simulink model "test_qdr_vacc2"  (Simulink 7.0)
settings: Solver=ode45  StartTime=0.0  StopTime=200000  RelTol=1e-3
libraries: xbsIndex_r4 x298, casper_library x21, xps_library x16
(part 1 of 3)
settings Model: Creator=Jason Manley  LastModifiedBy=dsp

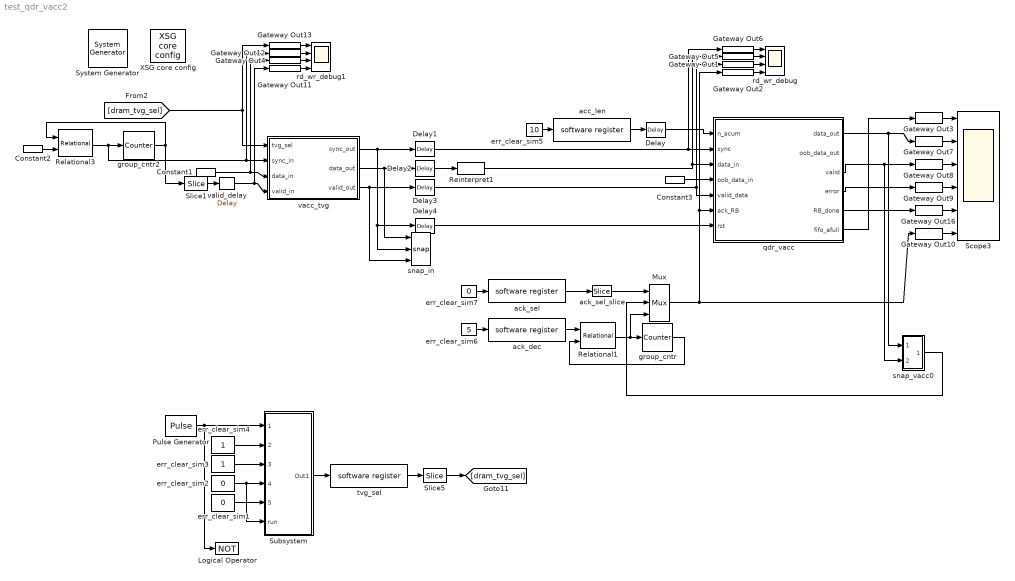
== system test_qdr_vacc2 ==
  " System Generator" : xbsIndex_r4/ System Generator  Tag=genX  SystemSampleTime=-1  xilinxfamily=virtex5  part=xc5vsx95t  speed=-1  package=ff1136  synthesis_tool=XST  clock_wrapper=Clock Enables  directory=./test_qdr_vacc2/sysgen  testbench=off  simulink_period=1  sysclk_period=4.7619  dcm_input_clock_period=100  incr_netlist=off  trim_vbits=Everywhere in SubSystem  dbl_ovrd=According to Block Masks  core_generation=According to Block Masks  run_coregen=off  deprecated_control=off  eval_field=0  block_type=sysgen
      settings: block_version=10.1.3
  Constant1 : xbsIndex_r4/Constant  arith_type=Unsigned  const=0  n_bits=32  bin_pt=0  explicit_period=on  period=1  equ=P=C  opselect=C  inp2=PCIN>>17  opr=+  inp1=P  carry=CIN  dbl_ovrd=off  block_type=constant
  Constant2 : xbsIndex_r4/Constant  arith_type=Unsigned  const=(10*2*2*1000) -1  n_bits=32  bin_pt=0  explicit_period=on  period=1  equ=P=C  opselect=C  inp2=PCIN>>17  opr=+  inp1=P  carry=CIN  dbl_ovrd=off  block_type=constant
  Constant3 : xbsIndex_r4/Constant  arith_type=Unsigned  const=0  n_bits=4  bin_pt=0  explicit_period=on  period=1  equ=P=C  opselect=C  inp2=PCIN>>17  opr=+  inp1=P  carry=CIN  dbl_ovrd=off  block_type=constant
  Delay : xbsIndex_r4/Delay  en=off  latency=1  dbl_ovrd=off  reg_retiming=on  block_type=delay
  Delay{1..4} (4 alike) : xbsIndex_r4/Delay  en=off  latency=2  dbl_ovrd=off  reg_retiming=on  block_type=delay
  Gateway Out{1..2,4..6,11..13} (8 alike) : xbsIndex_r4/Gateway Out  hdl_port=on  timing_constraint=None  locs_specified=off  LOCs={}  block_type=gatewayout
      settings: infoedit="Gateway out block.  Converts Xilinx fixed point inputs into ouputs of type Simulink integer, double, or fixed point.<P><P>Hardware notes:  In hardware these blocks become top level output ports or are discarded, depending on how they are configured."  xl_area=[0, 0, 0, 0, 0, 0, 0]  block_version=10.1.3
  Gateway Out{3,7..10,16} (6 alike) : xbsIndex_r4/Gateway Out  hdl_port=off  timing_constraint=None  locs_specified=off  LOCs={}  block_type=gatewayout
      settings: infoedit="Gateway out block.  Converts Xilinx fixed point inputs into ouputs of type Simulink integer, double, or fixed point.<P><P>Hardware notes:  In hardware these blocks become top level output ports or are discarded, depending on how they are configured."  xl_area=[0, 0, 0, 0, 0, 0, 0]  block_version=10.1.3
  Logical Operator : Logic  Operator=NOT  AllPortsSameDT=off  OutDataTypeMode=boolean
  Mux : xbsIndex_r4/Mux  inputs=2  en=off  latency=0  precision=Full  arith_type=Unsigned  n_bits=16  bin_pt=14  quantization=Truncate  overflow=Wrap  dbl_ovrd=off  block_type=mux
  Pulse Generator : DiscretePulseGenerator  Period=8*100*8  PhaseDelay=2
  Reinterpret1 : xbsIndex_r4/Reinterpret  force_arith_type=on  arith_type="Signed  (2's comp)"  force_bin_pt=on  bin_pt=0  block_type=reinterpret
      settings: infoedit="Changes signal type without altering the binary representation.   You can changed the signal between signed and unsigned, and relocate the binary point.<P><P>Hardware notes: In hardware this block costs nothing.<P><P>Example:  Suppose the input is 6 bits wide, signed, with 2 fractional bits, and the output is forced to unsigned with 0 fractional bits.  Then an input of -2.0 (1110.00 in binary 2's complement) becomes an output of 56 (111000 in binary)."  block_version=9.2.01
  Relational1 : xbsIndex_r4/Relational  mode=a<=b  en=off  latency=0  dbl_ovrd=off  block_type=relational
      settings: xl_area=[0, 0, 0, 0, 0, 0, 0]  block_version=10.1.3
  Relational3 : xbsIndex_r4/Relational  mode=a>=b  en=off  latency=0  dbl_ovrd=off  block_type=relational
      settings: xl_area=[0, 0, 0, 0, 0, 0, 0]  block_version=10.1.3
  Scope3 : Scope  NumInputPorts=6
      settings: YMin=0~7250~0~-1~-1~0  YMax=1~10000~1~1~1~1  SaveName=ScopeData2
  Slice1 : xbsIndex_r4/Slice  nbits=1  boolean_output=on  mode=Lower Bit Location + Width  bit1=0  base1=MSB of Input  bit0=0  base0=LSB of Input  dbl_ovrd=off  block_type=slice
      settings: infoedit="Extracts a given range of bits from each input sample and presents it at the output.  The output type is ordinarily unsigned with binary point at zero, but can be Boolean when the slice is one bit wide.<P><P>Hardware notes: In hardware this block costs nothing."  block_version=10.1.3
  Slice5 : xbsIndex_r4/Slice  nbits=6  boolean_output=off  mode=Lower Bit Location + Width  bit1=0  base1=MSB of Input  bit0=9  base0=LSB of Input  dbl_ovrd=off  block_type=slice
      settings: infoedit="Extracts a given range of bits from each input sample and presents it at the output.  The output type is ordinarily unsigned with binary point at zero, but can be Boolean when the slice is one bit wide.<P><P>Hardware notes: In hardware this block costs nothing."  block_version=10.1.3
  Subsystem : Subsystem
  XSG core config : xps_library/XSG core config  Tag=xps:xsg  SystemSampleTime=-1  hw_sys=ROACH:sx95t  ibob_linux=off  clk_src=arb_clk  iBOB_clk_src=sys_clk  BEE2_ctrl_clk_src=sys_clk  BEE2_usr_clk_src=sys_clk  ROACH_clk_src=arb_clk  CORR_clk_src=sys_clk  gpio_clk_io_group=iBOB:sma  gpio_clk_bit_index=0  clk_rate=210  sample_period=1  synthesis_tool=XST  mpc_type=powerpc440_ext
  acc_len : xps_library/software register  Tag=xps:sw_reg  SystemSampleTime=-1  io_dir=From Processor  arith_type=Unsigned  bitwidth=32  bin_pt=0  sample_period=1  gw_name=test_qdr_vacc2_acc_len_user_data_out
      link override qdr_vacc_tvg_sel_user_data_out: arith_type=Unsigned  n_bits=32  bin_pt=0  period=1
      link override test_qdr_vacc2_acc_len_user_data_out: arith_type=Unsigned  n_bits=32  bin_pt=0  period=1
      link override test_qdr_vacc_acc_len_user_data_out: arith_type=Unsigned  n_bits=32  bin_pt=0  period=1
      link override test_qdr_vacc_tvg_sel_user_data_out: arith_type=Unsigned  n_bits=32  bin_pt=0  period=1
  ack_dec : xps_library/software register  Tag=xps:sw_reg  SystemSampleTime=-1  io_dir=From Processor  arith_type=Unsigned  bitwidth=32  bin_pt=0  sample_period=1  gw_name=test_qdr_vacc2_ack_dec_user_data_out
      link override qdr_vacc_tvg_sel_user_data_out: arith_type=Unsigned  n_bits=32  bin_pt=0  period=1
      link override test_qdr_vacc2_ack_dec_user_data_out: arith_type=Unsigned  n_bits=32  bin_pt=0  period=1
      link override test_qdr_vacc_acc_len_user_data_out: arith_type=Unsigned  n_bits=32  bin_pt=0  period=1
      link override test_qdr_vacc_ack_dec_user_data_out: arith_type=Unsigned  n_bits=32  bin_pt=0  period=1
      link override test_qdr_vacc_tvg_sel_user_data_out: arith_type=Unsigned  n_bits=32  bin_pt=0  period=1
  ack_sel : xps_library/software register  Tag=xps:sw_reg  SystemSampleTime=-1  io_dir=From Processor  arith_type=Unsigned  bitwidth=32  bin_pt=0  sample_period=1  gw_name=test_qdr_vacc2_ack_sel_user_data_out
      link override qdr_vacc_tvg_sel_user_data_out: arith_type=Unsigned  n_bits=32  bin_pt=0  period=1
      link override test_qdr_vacc2_ack_sel_user_data_out: arith_type=Unsigned  n_bits=32  bin_pt=0  period=1
      link override test_qdr_vacc_acc_len_user_data_out: arith_type=Unsigned  n_bits=32  bin_pt=0  period=1
      link override test_qdr_vacc_ack_dec_user_data_out: arith_type=Unsigned  n_bits=32  bin_pt=0  period=1
      link override test_qdr_vacc_ack_sel_user_data_out: arith_type=Unsigned  n_bits=32  bin_pt=0  period=1
      link override test_qdr_vacc_tvg_sel_user_data_out: arith_type=Unsigned  n_bits=32  bin_pt=0  period=1
  ack_sel_slice : xbsIndex_r4/Slice  nbits=1  boolean_output=on  mode=Lower Bit Location + Width  bit1=0  base1=LSB of Input  bit0=0  base0=LSB of Input  dbl_ovrd=off  block_type=slice
      settings: infoedit="Extracts a given range of bits from each input sample and presents it at the output.  The output type is ordinarily unsigned with binary point at zero, but can be Boolean when the slice is one bit wide.<P><P>Hardware notes: In hardware this block costs nothing."  block_version=10.1.1
  err_clear_sim1 : Constant  Value=0  OutDataType=sfix(16)  OutScaling=2^0
  err_clear_sim2 : Constant  Value=0  OutDataType=sfix(16)  OutScaling=2^0
  err_clear_sim3 : Constant  OutDataType=sfix(16)  OutScaling=2^0
  err_clear_sim4 : Constant  OutDataType=sfix(16)  OutScaling=2^0
  err_clear_sim5 : Constant  Value=10  OutDataType=sfix(16)  OutScaling=2^0
  err_clear_sim6 : Constant  Value=5  OutDataType=sfix(16)  OutScaling=2^0
  err_clear_sim7 : Constant  Value=0  OutDataType=sfix(16)  OutScaling=2^0
  group_cntr : xbsIndex_r4/Counter  cnt_type=Free Running  cnt_to=1  operation=Up  start_count=0  cnt_by_val=1  arith_type=Unsigned  n_bits=32  bin_pt=0  load_pin=off  rst=on  en=off  explicit_period=on  period=1  dbl_ovrd=off  use_behavioral_HDL=off  use_rpm=on  implementation=Fabric  block_type=counter
      settings: xl_area=[0, 0, 0, 0, 0, 0, 0]
  group_cntr2 : xbsIndex_r4/Counter  cnt_type=Free Running  cnt_to=1  operation=Up  start_count=0  cnt_by_val=1  arith_type=Unsigned  n_bits=32  bin_pt=0  load_pin=off  rst=on  en=off  explicit_period=on  period=1  dbl_ovrd=off  use_behavioral_HDL=off  use_rpm=on  implementation=Fabric  block_type=counter
      settings: xl_area=[0, 0, 0, 0, 0, 0, 0]
  qdr_vacc : Subsystem  AncestorBlock=casper_library/Accumulators/qdr_vacc  mask{vector_len=1000}
      mask prompts: vector_len "Vector length??(# cycles)"
      mask help:
      | A vector accumulator for medium length vectors designed for ROACH's QDR memory.
      |
      | Originally designed for the packetised correlator, this block accepts input data of type Fix_32_0. OOB_data_in provides an extra 4 bits that are accumulated seperately (originally designed to keep track of how many "bad" values in a vector were accumulated).
      |
      | Minimum vector length is 2 * burst_length.
      | Minimum burst length is 10 (recommended default is 2^4=16).
      |
      | The vector length does not need to be a multiple of the burst length.
      mask init:
      | vector_bits = ceil(log2(vector_len));
      | burst_bits = 4;
      | burst_len = 2^burst_bits;
      | 
      | fmtstr = sprintf('Vector Length: %d', vector_len);
      | set_param(gcb, 'AttributesFormatString', fmtstr);
      settings: AttributesFormatString=Vector Length: 1000
  rd_wr_debug : Scope  NumInputPorts=4
      settings: YMin=-1~0~0~1  YMax=1~10000~1~1  SaveName=ScopeData3
  rd_wr_debug1 : Scope  NumInputPorts=4
      settings: YMin=-1~0~0~0  YMax=1~150~1~1  SaveName=ScopeData8
  snap_in : casper_library/Scopes/snap  SystemSampleTime=-1  nsamples=11
      link override addr/convert: arith_type=Unsigned  n_bits=32  bin_pt=0
      link override bram/convert_din: arith_type=Unsigned
      link override bram/mem/sim_data_in: arith_type=Unsigned
      link override bram/test_qdr_vacc2_snap_in_bram_data_out: arith_type=Unsigned
      link override bram/test_qdr_vacc_snap_in_bram_data_out: arith_type=Unsigned
      link override ctrl/test_qdr_vacc2_snap_in_ctrl_user_data_out: arith_type=Unsigned  n_bits=32  bin_pt=0  period=1
      link override ctrl/test_qdr_vacc_snap_in_ctrl_user_data_out: arith_type=Unsigned  n_bits=32  bin_pt=0  period=1
  snap_vacc0 : Subsystem  AncestorBlock=casper_library/Scopes/snap  mask(snap){nsamples=11}
      mask prompts: nsamples "No. of samples(2^?)"
      mask help:
      | The <i>snap</i> block provides a packaged solution to capturing data from
      | the FPGA fabric and making it accessible from the CPU.  The block comes in
      | 2 flavors: <i>snap</i> (which captures to a 32 bit wide Shared BRAM), and
      | <i>snap64</i> (which captures to 2x32 bit wide Shared BRAMs to effect a
      | 64 bit capture).
      mask Help: eval('xlWeb([getenv(''MLIB_ROOT''), ''\doc\htmlblocks\sys_snap\sys_snap.html''])')
  tvg_sel : xps_library/software register  Tag=xps:sw_reg  SystemSampleTime=-1  io_dir=From Processor  arith_type=Unsigned  bitwidth=32  bin_pt=0  sample_period=1  gw_name=test_qdr_vacc2_tvg_sel_user_data_out
      link override qdr_vacc_tvg_sel_user_data_out: arith_type=Unsigned  n_bits=32  bin_pt=0  period=1
      link override test_qdr_vacc2_tvg_sel_user_data_out: arith_type=Unsigned  n_bits=32  bin_pt=0  period=1
      link override test_qdr_vacc_tvg_sel_user_data_out: arith_type=Unsigned  n_bits=32  bin_pt=0  period=1
  vacc_tvg : Subsystem  mask{len=1000}
      mask prompts: len "Number of Vectors"
      mask init:
      | fmtstr = sprintf('Vector Length: %d', len);
      | set_param(gcb, 'AttributesFormatString', fmtstr);
      settings: AttributesFormatString=Vector Length: 1000
  valid_delay : xbsIndex_r4/Delay  en=off  latency=1  dbl_ovrd=off  reg_retiming=on  block_type=delay
  wires:
  [dram_tvg_sel] -> Gateway Out13/1, vacc_tvg/1(tvg_sel)
  Constant1/1 -> Gateway Out4/1, vacc_tvg/3(data_in)
  tvg_sel/1 -> Slice5/1
  Slice5/1 -> [dram_tvg_sel]
  err_clear_sim1/1 -> Subsystem/5(data_sel)
  err_clear_sim2/1 -> Subsystem/4(valid_sel), Subsystem/6(run)
  err_clear_sim3/1 -> Subsystem/3(inj_vector)
  err_clear_sim4/1 -> Subsystem/2(inj_counter)
  Subsystem/1(Out1) -> tvg_sel/1
  Pulse Generator/1 -> Subsystem/1(new_acc), Logical Operator/1
  Relational3/1 -> group_cntr2/1, Gateway Out12/1, vacc_tvg/2(sync_in)
  Constant2/1 -> Relational3/2
  group_cntr2/1 -> Relational3/1, Slice1/1
  Gateway Out13/1 -> rd_wr_debug1/1
  Gateway Out12/1 -> rd_wr_debug1/2
  Gateway Out4/1 -> rd_wr_debug1/3
  Gateway Out11/1 -> rd_wr_debug1/4
  valid_delay/1 -> Gateway Out11/1, vacc_tvg/4(valid_in)
  Slice1/1 -> valid_delay/1
  vacc_tvg/1(sync_out) -> snap_in/2, Delay4/1, Delay1/1
  vacc_tvg/2(data_out) -> snap_in/1, Delay2/1
  vacc_tvg/3(valid_out) -> snap_in/3, Delay3/1
  acc_len/1 -> Delay/1
  err_clear_sim5/1 -> acc_len/1
  Delay/1 -> qdr_vacc/1(n_acum)
  Constant3/1 -> qdr_vacc/4(oob_data_in)
  Gateway Out6/1 -> rd_wr_debug/1
  Gateway Out5/1 -> rd_wr_debug/2
  Gateway Out1/1 -> rd_wr_debug/3
  Gateway Out2/1 -> rd_wr_debug/4
  Reinterpret1/1 -> Gateway Out5/1, qdr_vacc/3(data_in)
  Relational1/1 -> group_cntr/1, Mux/3
  group_cntr/1 -> Relational1/2
  err_clear_sim6/1 -> ack_dec/1
  ack_dec/1 -> Relational1/1
  err_clear_sim7/1 -> ack_sel/1
  ack_sel/1 -> ack_sel_slice/1
  ack_sel_slice/1 -> Mux/1
  Gateway Out3/1 -> Scope3/1
  Gateway Out7/1 -> Scope3/2
  Gateway Out8/1 -> Scope3/3
  Gateway Out9/1 -> Scope3/4
  Gateway Out16/1 -> Scope3/5
  Gateway Out10/1 -> Scope3/6
  qdr_vacc/1(data_out) -> Gateway Out7/1, snap_vacc0/1(din)
  qdr_vacc/3(valid) -> Gateway Out8/1, snap_vacc0/2(we)
  qdr_vacc/5(RB_done) -> Gateway Out16/1
  qdr_vacc/4(error) -> Gateway Out9/1
  snap_vacc0/1(fetch) -> Mux/2
  qdr_vacc/6(fifo_afull) -> Gateway Out3/1
  Mux/1 -> Gateway Out2/1, qdr_vacc/6(ack_RB), Gateway Out10/1
  Delay1/1 -> Gateway Out6/1, qdr_vacc/2(sync)
  Delay2/1 -> Reinterpret1/1
  Delay3/1 -> Gateway Out1/1, qdr_vacc/5(valid_data)
  Delay4/1 -> qdr_vacc/7(rst)

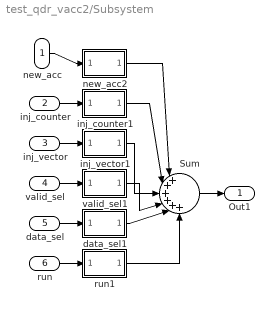
== system test_qdr_vacc2/Subsystem ==
  new_acc : Inport  OutDataType=sfix(16)  OutScaling=2^0
  inj_counter : Inport  Port=2  OutDataType=sfix(16)  OutScaling=2^0
  inj_vector : Inport  Port=3  OutDataType=sfix(16)  OutScaling=2^0
  valid_sel : Inport  Port=4  OutDataType=sfix(16)  OutScaling=2^0
  data_sel : Inport  Port=5  OutDataType=sfix(16)  OutScaling=2^0
  run : Inport  Port=6  OutDataType=sfix(16)  OutScaling=2^0
  Sum : Sum  Inputs=|++++++  OutDataType=sfix(16)  OutScaling=2^0
  data_sel1 : Subsystem  mask{bit_pos=10}
      mask prompts: bit_pos "bit position"
  inj_counter1 : Subsystem  mask{bit_pos=13}
      mask prompts: bit_pos "bit position"
  inj_vector1 : Subsystem  mask{bit_pos=12}
      mask prompts: bit_pos "bit position"
  new_acc2 : Subsystem  mask{bit_pos=14}
      mask prompts: bit_pos "bit position"
  run1 : Subsystem  mask{bit_pos=9}
      mask prompts: bit_pos "bit position"
  valid_sel1 : Subsystem  mask{bit_pos=11}
      mask prompts: bit_pos "bit position"
  Out1 : Outport  OutDataType=sfix(16)  OutScaling=2^0
  wires:
  new_acc2/1(Out1) -> Sum/1
  inj_counter1/1(Out1) -> Sum/2
  inj_vector1/1(Out1) -> Sum/3
  valid_sel1/1(Out1) -> Sum/4
  data_sel1/1(Out1) -> Sum/5
  run1/1(Out1) -> Sum/6
  new_acc/1 -> new_acc2/1(In1)
  inj_counter/1 -> inj_counter1/1(In1)
  inj_vector/1 -> inj_vector1/1(In1)
  valid_sel/1 -> valid_sel1/1(In1)
  Sum/1 -> Out1/1
  data_sel/1 -> data_sel1/1(In1)
  run/1 -> run1/1(In1)

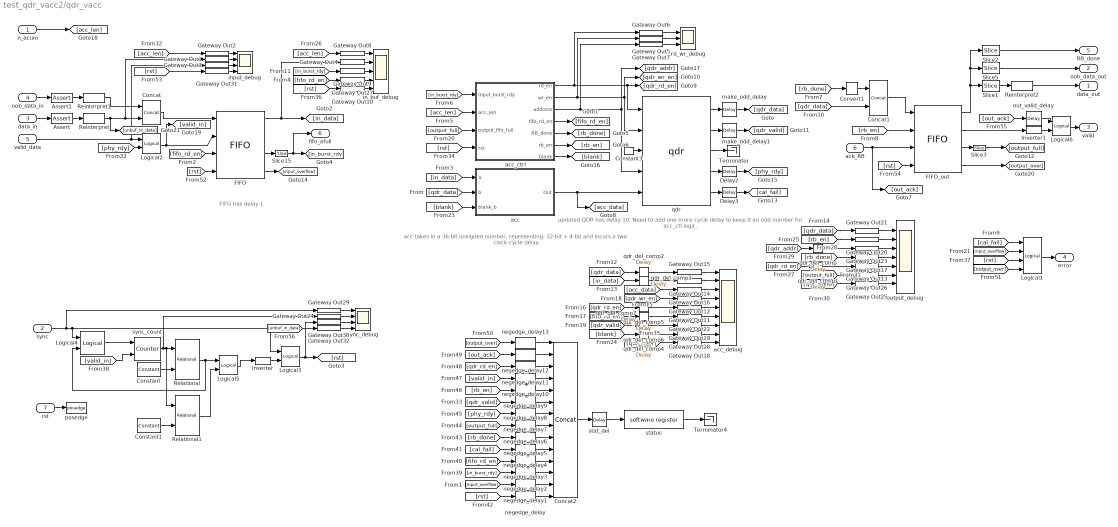
== system test_qdr_vacc2/qdr_vacc ==
  note: acc takes in a 36-bit unsigned
      | number, representing:
      | 32-bit + 4-bit and
      | incurs a two clock-cycle delay
  note: FIFO has delay 1
  note: updated QDR has delay 10.
      | Need to add one more cycle delay
      | to keep it an odd number for acc_ctl logic.
  n_acum : Inport  OutDataType=sfix(16)  OutScaling=2^0
  sync : Inport  Port=2  OutDataType=sfix(16)  OutScaling=2^0
  data_in : Inport  Port=3  OutDataType=sfix(16)  OutScaling=2^0
  oob_data_in : Inport  Port=4  OutDataType=sfix(16)  OutScaling=2^0
  valid_data : Inport  Port=5  OutDataType=sfix(16)  OutScaling=2^0
  ack_RB : Inport  Port=6  OutDataType=sfix(16)  OutScaling=2^0
  rst : Inport  Port=7  OutDataType=sfix(16)  OutScaling=2^0
  Assert : xbsIndex_r4/Assert  assert_type=on  type_source=Explicitly  arith_type="Signed  (2's comp)"  n_bits=32  bin_pt=0  assert_rate=off  rate_source=Explicitly  period=1  output_port=on  block_type=assert
      settings: infoedit=Asserts a user-defined sample rate and/or type on a signal.<P><P>Hardware notes: In hardware this block costs nothing.  block_version=10.1.3
  Assert1 : xbsIndex_r4/Assert  assert_type=on  type_source=Explicitly  arith_type=Unsigned  n_bits=4  bin_pt=0  assert_rate=on  rate_source=Explicitly  period=1  output_port=on  block_type=assert
      settings: infoedit=Asserts a user-defined sample rate and/or type on a signal.<P><P>Hardware notes: In hardware this block costs nothing.  block_version=10.1.3
  Concat : xbsIndex_r4/Concat  num_inputs=2  dbl_ovrd=off  block_type=concat
      settings: block_version=9.2.01
  Concat1 : xbsIndex_r4/Concat  num_inputs=2  dbl_ovrd=off  block_type=concat
      settings: block_version=9.2.01
  Concat2 : xbsIndex_r4/Concat  num_inputs=14  dbl_ovrd=off  block_type=concat
      settings: block_version=9.2.01
  Constant : xbsIndex_r4/Constant  arith_type=Unsigned  const=vector_len  n_bits=vector_bits  bin_pt=0  explicit_period=on  period=1  equ=P=C  opselect=C  inp2=PCIN>>17  opr=+  inp1=P  carry=CIN  dbl_ovrd=off  block_type=constant
  Constant1 : xbsIndex_r4/Constant  arith_type=Unsigned  const=0  n_bits=vector_bits  bin_pt=0  explicit_period=on  period=1  equ=P=C  opselect=C  inp2=PCIN>>17  opr=+  inp1=P  carry=CIN  dbl_ovrd=off  block_type=constant
  Constant3 : xbsIndex_r4/Constant  arith_type=Unsigned  const=(2^4)-1  n_bits=4  bin_pt=0  explicit_period=on  period=1  equ=P=C  opselect=C  inp2=PCIN>>17  opr=+  inp1=P  carry=CIN  dbl_ovrd=off  block_type=constant
      settings: block_version=9.2.01
  Convert1 : xbsIndex_r4/Convert  arith_type=Unsigned  n_bits=1  bin_pt=0  quantization=Truncate  overflow=Wrap  latency=0  dbl_ovrd=off  pipeline=off  block_type=convert
      settings: xl_area=[0, 0, 0, 0, 0, 0, 0]  block_version=9.2.01
  Delay2 : xbsIndex_r4/Delay  en=off  latency=2  dbl_ovrd=off  reg_retiming=on  block_type=delay
  Delay3 : xbsIndex_r4/Delay  en=off  latency=2  dbl_ovrd=off  reg_retiming=on  block_type=delay
  FIFO : xbsIndex_r4/FIFO  depth=64  percent_nbits=2  rst=on  en=off  use_dcount=off  use_almost_empty=off  almost_empty_thresh=2  use_almost_full=off  almost_full_thresh=14  dbl_ovrd=off  mem_type=Block RAM  block_type=fifo
      settings: block_version=10.1.3
  FIFO_out : xbsIndex_r4/FIFO  depth=512  percent_nbits=2  rst=on  en=off  use_dcount=off  use_almost_empty=off  almost_empty_thresh=2  use_almost_full=off  almost_full_thresh=14  dbl_ovrd=off  mem_type=Block RAM  block_type=fifo
      settings: block_version=10.1.3
  Gateway Out{1..32} (32 alike) : xbsIndex_r4/Gateway Out  hdl_port=off  timing_constraint=None  locs_specified=off  LOCs={}  block_type=gatewayout
      settings: infoedit="Gateway out block.  Converts Xilinx fixed point inputs into ouputs of type Simulink integer, double, or fixed point.<P><P>Hardware notes:  In hardware these blocks become top level output ports or are discarded, depending on how they are configured."  xl_area=[0, 0, 0, 0, 0, 0, 0]  block_version=10.1.3
  Inverter : xbsIndex_r4/Inverter  en=off  latency=0  dbl_ovrd=off  block_type=inv
  Inverter1 : xbsIndex_r4/Inverter  en=off  latency=0  dbl_ovrd=off  block_type=inv
  Logical1 : xbsIndex_r4/Logical  logical_function=OR  inputs=4  en=off  latency=1  precision=Full  arith_type=Unsigned  n_bits=16  bin_pt=0  align_bp=on  dbl_ovrd=off  block_type=logical
  Logical2 : xbsIndex_r4/Logical  logical_function=AND  inputs=2  en=off  latency=0  precision=Full  arith_type=Unsigned  n_bits=16  bin_pt=0  align_bp=on  dbl_ovrd=off  block_type=logical
  Logical3 : xbsIndex_r4/Logical  logical_function=AND  inputs=2  en=off  latency=0  precision=Full  arith_type=Unsigned  n_bits=16  bin_pt=0  align_bp=on  dbl_ovrd=off  block_type=logical
  Logical4 : xbsIndex_r4/Logical  logical_function=OR  inputs=2  en=off  latency=0  precision=Full  arith_type=Unsigned  n_bits=16  bin_pt=0  align_bp=on  dbl_ovrd=off  block_type=logical
  Logical5 : xbsIndex_r4/Logical  logical_function=OR  inputs=2  en=off  latency=0  precision=Full  arith_type=Unsigned  n_bits=16  bin_pt=0  align_bp=on  dbl_ovrd=off  block_type=logical
  Logical6 : xbsIndex_r4/Logical  logical_function=AND  inputs=2  en=off  latency=0  precision=Full  arith_type=Unsigned  n_bits=16  bin_pt=0  align_bp=on  dbl_ovrd=off  block_type=logical
  Reinterpret : xbsIndex_r4/Reinterpret  force_arith_type=on  arith_type=Unsigned  force_bin_pt=on  bin_pt=0  block_type=reinterpret
      settings: infoedit="Changes signal type without altering the binary representation.   You can changed the signal between signed and unsigned, and relocate the binary point.<P><P>Hardware notes: In hardware this block costs nothing.<P><P>Example:  Suppose the input is 6 bits wide, signed, with 2 fractional bits, and the output is forced to unsigned with 0 fractional bits.  Then an input of -2.0 (1110.00 in binary 2's complement) becomes an output of 56 (111000 in binary)."  block_version=9.2.01
  Reinterpret1 : xbsIndex_r4/Reinterpret  force_arith_type=on  arith_type=Unsigned  force_bin_pt=on  bin_pt=0  block_type=reinterpret
      settings: infoedit="Changes signal type without altering the binary representation.   You can changed the signal between signed and unsigned, and relocate the binary point.<P><P>Hardware notes: In hardware this block costs nothing.<P><P>Example:  Suppose the input is 6 bits wide, signed, with 2 fractional bits, and the output is forced to unsigned with 0 fractional bits.  Then an input of -2.0 (1110.00 in binary 2's complement) becomes an output of 56 (111000 in binary)."  block_version=9.2.01
  Reinterpret2 : xbsIndex_r4/Reinterpret  force_arith_type=on  arith_type="Signed  (2's comp)"  force_bin_pt=on  bin_pt=0  block_type=reinterpret
      settings: infoedit="Changes signal type without altering the binary representation.   You can changed the signal between signed and unsigned, and relocate the binary point.<P><P>Hardware notes: In hardware this block costs nothing.<P><P>Example:  Suppose the input is 6 bits wide, signed, with 2 fractional bits, and the output is forced to unsigned with 0 fractional bits.  Then an input of -2.0 (1110.00 in binary 2's complement) becomes an output of 56 (111000 in binary)."  block_version=9.2.01
  Relational : xbsIndex_r4/Relational  mode=a>=b  en=off  latency=0  dbl_ovrd=off  block_type=relational
      settings: block_version=10.1.3
  Relational1 : xbsIndex_r4/Relational  mode=a=b  en=off  latency=0  dbl_ovrd=off  block_type=relational
      settings: block_version=10.1.3
  Slice1 : xbsIndex_r4/Slice  nbits=32  boolean_output=off  mode=Lower Bit Location + Width  bit1=96  base1=MSB of Input  bit0=0  base0=LSB of Input  dbl_ovrd=off  block_type=slice
      settings: infoedit="Extracts a given range of bits from each input sample and presents it at the output.  The output type is ordinarily unsigned with binary point at zero, but can be Boolean when the slice is one bit wide.<P><P>Hardware notes: In hardware this block costs nothing."  block_version=9.2.01
  Slice15 : xbsIndex_r4/Slice  nbits=1  boolean_output=on  mode=Upper Bit Location + Width  bit1=0  base1=MSB of Input  bit0=0  base0=LSB of Input  dbl_ovrd=off  block_type=slice
      settings: infoedit="Extracts a given range of bits from each input sample and presents it at the output.  The output type is ordinarily unsigned with binary point at zero, but can be Boolean when the slice is one bit wide.<P><P>Hardware notes: In hardware this block costs nothing."  block_version=9.2.01
  Slice2 : xbsIndex_r4/Slice  nbits=1  boolean_output=on  mode=Lower Bit Location + Width  bit1=-1  base1=MSB of Input  bit0=36  base0=LSB of Input  dbl_ovrd=off  block_type=slice
      settings: infoedit="Extracts a given range of bits from each input sample and presents it at the output.  The output type is ordinarily unsigned with binary point at zero, but can be Boolean when the slice is one bit wide.<P><P>Hardware notes: In hardware this block costs nothing."  block_version=9.2.01
  Slice3 : xbsIndex_r4/Slice  nbits=1  boolean_output=on  mode=Upper Bit Location + Width  bit1=0  base1=MSB of Input  bit0=0  base0=LSB of Input  dbl_ovrd=off  block_type=slice
      settings: infoedit="Extracts a given range of bits from each input sample and presents it at the output.  The output type is ordinarily unsigned with binary point at zero, but can be Boolean when the slice is one bit wide.<P><P>Hardware notes: In hardware this block costs nothing."  block_version=9.2.01
  Slice5 : xbsIndex_r4/Slice  nbits=4  boolean_output=off  mode=Lower Bit Location + Width  bit1=96  base1=MSB of Input  bit0=32  base0=LSB of Input  dbl_ovrd=off  block_type=slice
      settings: infoedit="Extracts a given range of bits from each input sample and presents it at the output.  The output type is ordinarily unsigned with binary point at zero, but can be Boolean when the slice is one bit wide.<P><P>Hardware notes: In hardware this block costs nothing."  block_version=9.2.01
  Terminator : Terminator
  Terminator4 : Terminator
  acc : Subsystem
  acc_ctrl : Subsystem  mask{delay_qdr=11, delay_in_fifo=1, delay_adder=2}
      mask prompts: delay_qdr "delay qdr"
      mask help: QDR delay must be odd (9 is ok, 11 is ok, 10 is not).
  acc_debug : Scope  NumInputPorts=9
      settings: TimeRange=57000  YMin=0~0~0~0~0~0~0~0~0  YMax=5e+009~1000~5e+009~1~1~1~1~1~1250  SaveName=ScopeData4
  in_buf_debug : Scope  NumInputPorts=5
      settings: YMin=7.6~-1~-1~-1~-1  YMax=8.4~1~1~1~1  SaveName=ScopeData2
  input_debug : Scope  NumInputPorts=4
      settings: YMin=12000~0~-5~-5  YMax=13300~1~5~5
  make_odd_delay : xbsIndex_r4/Delay  en=off  latency=1  dbl_ovrd=off  reg_retiming=on  block_type=delay
  make_odd_delay1 : xbsIndex_r4/Delay  en=off  latency=1  dbl_ovrd=off  reg_retiming=on  block_type=delay
  negedge_delay{,1..13} (14 alike) : casper_library/Misc/negedge_delay  SystemSampleTime=-1  pulse_len=2^23
  out_valid_delay : xbsIndex_r4/Delay  en=off  latency=1  dbl_ovrd=off  reg_retiming=on  block_type=delay
  output_debug : Scope  NumInputPorts=7
      settings: YMin=0~0~0~0~0~0~0  YMax=4.5e+009~1~1250~1~1~1~1  SaveName=ScopeData3
  posedge : casper_library/Misc/posedge  Tag=Rising Edge Detector  SystemSampleTime=-1
  qdr : xps_library/qdr  Tag=xps:qdr  SystemSampleTime=-1  which_qdr=qdr0  qdr_awidth=13  use_sniffer=on
  qdr_del_comp : xbsIndex_r4/Delay  en=off  latency=11  dbl_ovrd=off  reg_retiming=on  block_type=delay
  qdr_del_comp1 : xbsIndex_r4/Delay  en=off  latency=11  dbl_ovrd=off  reg_retiming=on  block_type=delay
  qdr_del_comp{2..4,6} (4 alike) : xbsIndex_r4/Delay  en=off  latency=2  dbl_ovrd=off  reg_retiming=on  block_type=delay
  qdr_del_comp5 : xbsIndex_r4/Delay  en=off  latency=13  dbl_ovrd=off  reg_retiming=on  block_type=delay
  qdr_del_comp7 : xbsIndex_r4/Delay  en=off  latency=3  dbl_ovrd=off  reg_retiming=on  block_type=delay
  rd_wr_debug : Scope  NumInputPorts=3
      settings: YMin=0~0~0  YMax=1~1~1050
  stat_del : xbsIndex_r4/Delay  en=off  latency=1  dbl_ovrd=off  reg_retiming=on  block_type=delay
  status : xps_library/software register  Tag=xps:sw_reg  SystemSampleTime=-1  io_dir=To Processor  arith_type=Unsigned  bitwidth=32  bin_pt=0  sample_period=1  gw_name=test_qdr_vacc2_qdr_vacc_status_user_data_in
      link override convert: arith_type=Unsigned  n_bits=32  bin_pt=0
  sync_count : xbsIndex_r4/Counter  cnt_type=Free Running  cnt_to=Inf  operation=Up  start_count=0  cnt_by_val=1  arith_type=Unsigned  n_bits=vector_bits  bin_pt=0  load_pin=off  rst=on  en=on  explicit_period=on  period=1  dbl_ovrd=off  use_behavioral_HDL=on  use_rpm=on  implementation=Fabric  block_type=counter
  sync_debug : Scope  NumInputPorts=4
      settings: YMin=-1~0~-1~0  YMax=1~1000~1~10000  SaveName=ScopeData2
  data_out : Outport  OutDataType=sfix(16)  OutScaling=2^0
  oob_data_out : Outport  Port=2  OutDataType=sfix(16)  OutScaling=2^0
  valid : Outport  Port=3  OutDataType=sfix(16)  OutScaling=2^0
  error : Outport  Port=4  OutDataType=sfix(16)  OutScaling=2^0
  RB_done : Outport  Port=5  OutDataType=sfix(16)  OutScaling=2^0
  fifo_afull : Outport  Port=6  OutDataType=sfix(16)  OutScaling=2^0
  wires:
  qdr_del_comp1/1 -> Gateway Out13/1
  qdr_del_comp/1 -> Gateway Out23/1
  make_odd_delay1/1 -> [qdr_valid]
  make_odd_delay/1 -> [qdr_data]
  Inverter/1 -> Logical3/2
  Logical3/1 -> [rst], Gateway Out30/1
  sync/1 -> Logical3/1, Logical4/1, Gateway Out29/1
  Reinterpret1/1 -> Concat/1
  Reinterpret/1 -> Gateway Out1/1, Concat/2, [unbuf_in_data]
  Assert1/1 -> Reinterpret1/1
  Assert/1 -> Reinterpret/1
  [in_data] -> acc/1(a)
  rst/1 -> posedge/1
  [rst] -> Gateway Out10/1
  Gateway Out10/1 -> in_buf_debug/5
  Gateway Out18/1 -> acc_debug/9
  [qdr_addr] -> Gateway Out18/1
  [rst] -> acc_ctrl/4(rst)
  [acc_len] -> Gateway Out2/1
  [acc_len] -> Gateway Out8/1
  [acc_len] -> acc_ctrl/2(acc_len)
  oob_data_in/1 -> Assert1/1
  n_acum/1 -> [acc_len]
  Gateway Out23/1 -> output_debug/3
  [qdr_addr] -> qdr_del_comp/1
  Gateway Out26/1 -> output_debug/6
  [rb_done] -> Gateway Out17/1
  [rb_en] -> Gateway Out20/1
  Gateway Out25/1 -> output_debug/7
  Gateway Out13/1 -> output_debug/5
  Gateway Out17/1 -> output_debug/4
  Gateway Out20/1 -> output_debug/2
  Gateway Out21/1 -> output_debug/1
  [output_full] -> Gateway Out26/1
  [qdr_valid] -> Gateway Out25/1
  [qdr_rd_en] -> qdr_del_comp1/1
  [qdr_data] -> Gateway Out21/1
  Gateway Out28/1 -> acc_debug/8
  Gateway Out19/1 -> acc_debug/7
  Gateway Out22/1 -> acc_debug/6
  Gateway Out11/1 -> acc_debug/5
  Gateway Out12/1 -> acc_debug/4
  Gateway Out16/1 -> acc_debug/3
  Gateway Out14/1 -> acc_debug/2
  Gateway Out15/1 -> acc_debug/1
  [blank] -> qdr_del_comp4/1
  [blank] -> acc/3(blank_b)
  acc_ctrl/7(blank) -> [blank]
  [qdr_data] -> acc/2(b)
  FIFO_out/4 -> [output_over]
  qdr/3 -> Terminator/1
  [phy_rdy] -> Logical2/2
  Logical2/1 -> [valid_in], FIFO/2
  Delay3/1 -> [cal_fail]
  Delay2/1 -> [phy_rdy]
  qdr/4 -> Delay2/1
  FIFO/4 -> [input_overflow]
  qdr/5 -> Delay3/1
  Logical1/1 -> error/1
  acc_ctrl/5(RB_done) -> [rb_done]
  acc_ctrl/6(rb_en) -> [rb_en]
  FIFO_out/3 -> Slice3/1
  [output_full] -> acc_ctrl/3(output_fifo_full)
  [qdr_valid] -> qdr_del_comp6/1
  qdr/2 -> make_odd_delay1/1
  [qdr_wr_en] -> Gateway Out12/1
  [fifo_rd_en] -> qdr_del_comp7/1
  [qdr_rd_en] -> qdr_del_comp5/1
  [acc_data] -> Gateway Out16/1
  [in_data] -> qdr_del_comp3/1
  [qdr_data] -> qdr_del_comp2/1
  Slice5/1 -> oob_data_out/1
  [in_burst_rdy] -> Gateway Out9/1
  [fifo_rd_en] -> Gateway Out27/1
  Gateway Out27/1 -> in_buf_debug/4
  Gateway Out9/1 -> in_buf_debug/3
  Gateway Out4/1 -> in_buf_debug/2
  Gateway Out8/1 -> in_buf_debug/1
  Gateway Out3/1 -> input_debug/3
  Gateway Out1/1 -> input_debug/2
  Gateway Out2/1 -> input_debug/1
  acc/1(Out) -> qdr/5, [acc_data]
  Gateway Out7/1 -> rd_wr_debug/3
  Gateway Out5/1 -> rd_wr_debug/2
  Gateway Out6/1 -> rd_wr_debug/1
  Slice1/1 -> Reinterpret2/1
  Slice2/1 -> RB_done/1
  FIFO_out/1 -> Slice5/1, Slice2/1, Slice1/1
  Convert1/1 -> Concat1/1
  [rb_done] -> Convert1/1
  Concat1/1 -> FIFO_out/1
  [qdr_data] -> Concat1/2
  [rb_en] -> FIFO_out/2
  ack_RB/1 -> [out_ack], FIFO_out/3
  [out_ack] -> out_valid_delay/1
  Slice15/1 -> [in_burst_rdy], fifo_afull/1
  [in_burst_rdy] -> acc_ctrl/1(input_burst_rdy)
  FIFO/1 -> Gateway Out4/1, [in_data]
  acc_ctrl/4(fifo_rd_en) -> [fifo_rd_en]
  Constant3/1 -> qdr/3
  qdr/1 -> make_odd_delay/1
  acc_ctrl/3(address) -> Gateway Out7/1, qdr/4, [qdr_addr]
  acc_ctrl/2(wr_en) -> Gateway Out5/1, qdr/2, [qdr_wr_en]
  acc_ctrl/1(rd_en) -> Gateway Out6/1, qdr/1, [qdr_rd_en]
  Concat/1 -> FIFO/1
  valid_data/1 -> Logical2/1, Gateway Out3/1
  data_in/1 -> Assert/1
  Constant/1 -> Relational/2
  Logical4/1 -> sync_count/1
  Relational/1 -> Logical4/2, Logical5/1
  sync_count/1 -> Gateway Out24/1, Relational/1, Relational1/1
  Gateway Out30/1 -> sync_debug/3
  Gateway Out24/1 -> sync_debug/2
  Gateway Out29/1 -> sync_debug/1
  [valid_in] -> sync_count/2
  Constant1/1 -> Relational1/2
  Logical5/1 -> Inverter/1
  Relational1/1 -> Logical5/2
  FIFO/3 -> Slice15/1
  [rst] -> negedge_delay/1
  [input_overflow] -> negedge_delay1/1
  [in_burst_rdy] -> negedge_delay2/1
  [fifo_rd_en] -> negedge_delay3/1
  [cal_fail] -> negedge_delay4/1
  [rb_done] -> negedge_delay5/1
  [output_full] -> negedge_delay6/1
  [phy_rdy] -> negedge_delay7/1
  Concat2/1 -> stat_del/1
  status/1 -> Terminator4/1
  stat_del/1 -> status/1
  [qdr_valid] -> negedge_delay8/1
  [valid_in] -> negedge_delay10/1
  [rb_en] -> negedge_delay9/1
  [qdr_rd_en] -> negedge_delay11/1
  [out_ack] -> negedge_delay12/1
  [output_over] -> negedge_delay13/1
  [cal_fail] -> Logical1/1
  [input_overflow] -> Logical1/2
  [rst] -> Logical1/3
  [output_over] -> Logical1/4
  negedge_delay13/1 -> Concat2/1
  negedge_delay12/1 -> Concat2/2
  negedge_delay11/1 -> Concat2/3
  negedge_delay10/1 -> Concat2/4
  negedge_delay9/1 -> Concat2/5
  negedge_delay8/1 -> Concat2/6
  negedge_delay7/1 -> Concat2/7
  negedge_delay6/1 -> Concat2/8
  negedge_delay5/1 -> Concat2/9
  negedge_delay4/1 -> Concat2/10
  negedge_delay3/1 -> Concat2/11
  negedge_delay2/1 -> Concat2/12
  negedge_delay1/1 -> Concat2/13
  negedge_delay/1 -> Concat2/14
  [rst] -> FIFO/4
  Reinterpret2/1 -> data_out/1
  Gateway Out31/1 -> input_debug/4
  [rst] -> Gateway Out31/1
  [rst] -> FIFO_out/4
  Inverter1/1 -> Logical6/2
  out_valid_delay/1 -> Logical6/1
  FIFO_out/2 -> Inverter1/1
  Logical6/1 -> valid/1
  Slice3/1 -> [output_full]
  qdr_del_comp2/1 -> Gateway Out15/1
  qdr_del_comp3/1 -> Gateway Out14/1
  qdr_del_comp4/1 -> Gateway Out28/1
  qdr_del_comp5/1 -> Gateway Out11/1
  qdr_del_comp6/1 -> Gateway Out19/1
  qdr_del_comp7/1 -> Gateway Out22/1
  Gateway Out32/1 -> sync_debug/4
  [unbuf_in_data] -> Gateway Out32/1
  [fifo_rd_en] -> FIFO/3

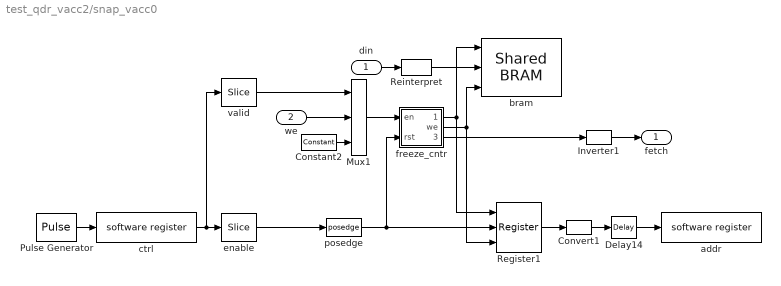
== system test_qdr_vacc2/snap_vacc0 ==
  din : Inport  OutDataType=sfix(16)  OutScaling=2^0
  we : Inport  Port=2  OutDataType=sfix(16)  OutScaling=2^0
  Constant2 : xbsIndex_r4/Constant  arith_type=Boolean  const=1  n_bits=1  bin_pt=0  explicit_period=on  period=1  equ=P=C  opselect=C  inp2=PCIN>>17  opr=+  inp1=P  carry=CIN  dbl_ovrd=off  block_type=constant
      settings: block_version=10.1.1
  Convert1 : xbsIndex_r4/Convert  arith_type=Unsigned  n_bits=32  bin_pt=0  quantization=Truncate  overflow=Wrap  latency=0  dbl_ovrd=off  pipeline=off  block_type=convert
      settings: block_version=10.1.3
  Delay14 : xbsIndex_r4/Delay  en=off  latency=1  dbl_ovrd=off  reg_retiming=on  block_type=delay
      settings: xl_area=[0, 0, 0, 0, 0, 0, 0]
  Inverter1 : xbsIndex_r4/Inverter  en=off  latency=0  dbl_ovrd=off  block_type=inv
      settings: xl_area=[0, 0, 0, 0, 0, 0, 0]
  Mux1 : xbsIndex_r4/Mux  inputs=2  en=off  latency=0  precision=Full  arith_type="Signed  (2's comp)"  n_bits=8  bin_pt=2  quantization=Truncate  overflow=Wrap  dbl_ovrd=off  block_type=mux
      settings: xl_area=[0, 0, 0, 0, 0, 0, 0]  block_version=10.1.1
  Pulse Generator : DiscretePulseGenerator  Period=(2*2*1000)  PhaseDelay=5
  Register1 : xbsIndex_r4/Register  init=0  rst=on  en=on  dbl_ovrd=off  block_type=register
      settings: xl_area=[0, 0, 0, 0, 0, 0, 0]  block_version=10.1.1
  Reinterpret : xbsIndex_r4/Reinterpret  force_arith_type=on  arith_type=Unsigned  force_bin_pt=on  bin_pt=0  block_type=reinterpret
      settings: infoedit="Changes signal type without altering the binary representation.   You can changed the signal between signed and unsigned, and relocate the binary point.<P><P>Hardware notes: In hardware this block costs nothing.<P><P>Example:  Suppose the input is 6 bits wide, signed, with 2 fractional bits, and the output is forced to unsigned with 0 fractional bits.  Then an input of -2.0 (1110.00 in binary 2's complement) becomes an output of 56 (111000 in binary)."  block_version=10.1.1
  addr : xps_library/software register  Tag=xps:sw_reg  SystemSampleTime=-1  io_dir=To Processor  arith_type=Unsigned  bitwidth=32  bin_pt=0  sample_period=1  gw_name=test_qdr_vacc2_snap_vacc0_addr_user_data_in
      link override convert: arith_type=Unsigned  n_bits=32  bin_pt=0
  bram : xps_library/Shared BRAM  Tag=xps:bram  SystemSampleTime=-1  arith_type=Unsigned  addr_width=nsamples  data_width=32  data_bin_pt=0  init_vals=0  sample_rate=1
      link override convert_din: arith_type=Unsigned
      link override mem/sim_data_in: arith_type=Unsigned
      link override r_4f_1x_16a_r322h_snap_xeng0_bram_data_out: arith_type=Unsigned
      link override r_4f_1x_16a_r322i_snap_xeng0_bram_data_out: arith_type=Unsigned
      link override r_4f_1x_16a_r322j_snap_xeng0_bram_data_out: arith_type=Unsigned
      link override r_4f_2x_16a_r322d_snap_descramble0_bram_data_out: arith_type=Unsigned
      link override r_4f_2x_16a_r322e_snap_descramble0_bram_data_out: arith_type=Unsigned
      link override r_4f_2x_16a_r322e_snap_xeng0_bram_data_out: arith_type=Unsigned
      link override r_4f_2x_16a_r322f_snap_xeng0_bram_data_out: arith_type=Unsigned
      link override r_4f_2x_16a_r322g_snap_xeng0_bram_data_out: arith_type=Unsigned
      link override r_4f_2x_16a_r322h_snap_xeng0_bram_data_out: arith_type=Unsigned
      link override test_qdr_vacc2_snap_vacc0_bram_data_out: arith_type=Unsigned
      link override test_snap2_10_1_snap_circ_bram_lsb_data_out: arith_type=Unsigned
  ctrl : xps_library/software register  Tag=xps:sw_reg  SystemSampleTime=-1  io_dir=From Processor  arith_type=Unsigned  bitwidth=32  bin_pt=0  sample_period=1  gw_name=test_qdr_vacc2_snap_vacc0_ctrl_user_data_out
      link override r_4f_1x_16a_r322k_snap_vacc0_ctrl_user_data_out: arith_type=Unsigned  n_bits=32  bin_pt=0  period=1
      link override test_qdr_vacc2_snap_vacc0_ctrl_user_data_out: arith_type=Unsigned  n_bits=32  bin_pt=0  period=1
      link override test_qdr_vacc_snap_vacc0_ctrl_user_data_out: arith_type=Unsigned  n_bits=32  bin_pt=0  period=1
  enable : xbsIndex_r4/Slice  nbits=1  boolean_output=on  mode=Lower Bit Location + Width  bit1=0  base1=LSB of Input  bit0=0  base0=LSB of Input  dbl_ovrd=off  block_type=slice
      settings: infoedit="Extracts a given range of bits from each input sample and presents it at the output.  The output type is ordinarily unsigned with binary point at zero, but can be Boolean when the slice is one bit wide.<P><P>Hardware notes: In hardware this block costs nothing."  block_version=10.1.1
  freeze_cntr : Subsystem  AncestorBlock=casper_library/Misc/freeze_cntr  mask(freeze_cntr){CounterBits=nsamples}
      mask prompts: CounterBits "Counter Length (2^?)"
      mask help:
      | A freeze counter is an enabled counter which holds its final value (regardless of enables)
      | until it is reset.
      mask Help: eval('xlWeb([getenv(''MLIB_ROOT''), ''\doc\htmlblocks\sp_freeze_cntr\sp_freeze_cntr.html''])')
  posedge : casper_library/Misc/posedge  Tag=Rising Edge Detector  SystemSampleTime=-1
  valid : xbsIndex_r4/Slice  nbits=1  boolean_output=on  mode=Lower Bit Location + Width  bit1=0  base1=LSB of Input  bit0=2  base0=LSB of Input  dbl_ovrd=off  block_type=slice
      settings: infoedit="Extracts a given range of bits from each input sample and presents it at the output.  The output type is ordinarily unsigned with binary point at zero, but can be Boolean when the slice is one bit wide.<P><P>Hardware notes: In hardware this block costs nothing."  block_version=10.1.1
  fetch : Outport  OutDataType=sfix(16)  OutScaling=2^0
  wires:
  valid/1 -> Mux1/1
  Constant2/1 -> Mux1/3
  we/1 -> Mux1/2
  Mux1/1 -> freeze_cntr/1(en)
  posedge/1 -> Register1/2, freeze_cntr/2(rst)
  ctrl/1 -> enable/1, valid/1
  din/1 -> Reinterpret/1
  Reinterpret/1 -> bram/2
  Pulse Generator/1 -> ctrl/1
  freeze_cntr/2(we) -> Register1/3, bram/3
  enable/1 -> posedge/1
  freeze_cntr/1(addr) -> Register1/1, bram/1
  Convert1/1 -> Delay14/1
  Delay14/1 -> addr/1
  freeze_cntr/3(afull) -> Inverter1/1
  Inverter1/1 -> fetch/1
  Register1/1 -> Convert1/1
